simulink model "EcoSIM3_P2_C2"  (R2014b)
settings: Solver=ode1  SolverMode=SingleTasking  StartTime=0.0  StopTime=inf  FixedStep=0.01  RelTol=1e-3
PostLoadFcn:
  | %, if any(exist('dsrtsu_mdlpostloadfcn', 'file') == [2, 3, 6]), try dsrtsu_mdlpostloadfcn('Execute', bdroot); catch fprintf('Error in PostLoadFcn (dsrtsu_mdlpostloadfcn) for model "%s":\n %s\n', bdroot, lasterr); end, end,
InitFcn:
  | tic
  | %Startup_EcoSIM
values from neighbouring files (symbols this model uses):
  EngPwr = [0 5	10	15	20	25	30	35	40	45	50	55	60	65	70	75	80	85	90	95	100	105	110	115]    [Series_Maps.m]
  EngSpd = [0 477.4645 954.929 1909.858 2864.787 3819.716 4774.645 5729.574 6684.503]    [Series_Maps.m]
  EngTrq = [0	0	0	0	0	0	0	0	0	0	0	0	0	0	0	0	0	0	0	0	0	0	0	0 ... (first row only)    [Series_Maps.m]
  Power = [0 5 10 15 20 25 30]    [Series_Maps.m]
  Torque = [-50,-40,-30,-25,-20,-15,-10,-8,-6,-4,-2,0]    [Series_Maps.m]
undefined symbols (not defined in the file or in its folder): canChannel, Controls, DriveCycles, Driver, EM_EFF_MAP, EM_PwrLoss_MAP, Glbl, Plants, Veh_Dynamics
libraries: canmsglib x100, canlib x87, fl_lib x78, simulink x59, nesl_utility x40, sdl_lib x17, dspsigops x5, dspswit3 x3, dspstat3 x2, commnoisgen2 x1, dspfdesign x1
(part 6 of 15)

== system EcoSIM3_P2_C2/Supervisory Controller/Mode Operation/Accessory/ESS_Messages ==
  Bus Creator2 : BusCreator
  Constant : Constant
  Constant1 : Constant
  Constant2 : Constant
  Constant3 : Constant  Value=0
  Out1 : Outport
  wires:
  Constant/1 -> Bus Creator2/3  "hsc_bcm_leakage_ena"
  Constant2/1 -> Bus Creator2/1  "hsc_bcm_enable"
  Constant1/1 -> Bus Creator2/2  "hsc_bcm_mainc_close"
  Bus Creator2/1 -> Out1/1  "ESS_Signals_A123"
  Constant3/1 -> Bus Creator2/4  "hsc_bcm_epo"

== system EcoSIM3_P2_C2/Supervisory Controller/Mode Operation/Accessory/Engine Messages ==
  Bus Creator2 : BusCreator  Inputs=3
  Constant1 : Constant  Value=0
  Constant2 : Constant  Value=0
  Constant3 : Constant  Value=0
  Out1 : Outport
  wires:
  Constant1/1 -> Bus Creator2/1  "ICE_Torque_Request_Nm"
  Constant2/1 -> Bus Creator2/2  "Engine_On"
  Constant3/1 -> Bus Creator2/3  "Engine_Run"
  Bus Creator2/1 -> Out1/1  "ICE_Request"

== system EcoSIM3_P2_C2/Supervisory Controller/Mode Operation/Accessory/TM Messages ==
  Bus Creator3 : BusCreator  Inputs=3
  Constant1 : Constant  Value=0
  Constant3 : Constant  Value=0
  Constant6 : Constant  Value=0
  Out1 : Outport
  wires:
  Bus Creator3/1 -> Out1/1  "EM_Messages_Rhinehart"
  Constant1/1 -> Bus Creator3/1  "Inverter_Enable"
  Constant6/1 -> Bus Creator3/2  "Torque_Command"
  Constant3/1 -> Bus Creator3/3  "Rotation_Direction"

== system EcoSIM3_P2_C2/Supervisory Controller/Mode Operation/Accessory/Trans_Messages ==
  Bus Creator3 : BusCreator  Inputs=2
  Constant8 : Constant  Value=0
  Constant9 : Constant  Value=0
  Out1 : Outport
  wires:
  Constant9/1 -> Bus Creator3/2  "Gear_Request"
  Constant8/1 -> Bus Creator3/1  "Shift_Request"
  Bus Creator3/1 -> Out1/1  "Trans_Recieve"

== system EcoSIM3_P2_C2/Supervisory Controller/Mode Operation/Charging/BAS_Signals ==
  Bus Creator4 : BusCreator  Inputs=3
  Constant1 : Constant  Value=0
  Constant4 : Constant  Value=0
  Constant5 : Constant  Value=0
  Out1 : Outport
  wires:
  Constant5/1 -> Bus Creator4/3  "BAS_Mode_Request"
  Constant4/1 -> Bus Creator4/1  "BAS_Torque_Request_Nm"
  Bus Creator4/1 -> Out1/1  "BAS_SoftECU_Receive"
  Constant1/1 -> Bus Creator4/2  "BAS_Speed_Request"

== system EcoSIM3_P2_C2/Supervisory Controller/Mode Operation/Charging/DC//DC Enabled ==
  Bus Creator : BusCreator  Inputs=3
  Constant : Constant
  Constant1 : Constant  Value=12.8
  Constant2 : Constant
  Out1 : Outport
  wires:
  Constant/1 -> Bus Creator/1  "LowVoltEnablRq"
  Constant1/1 -> Bus Creator/2  "LwVltStpntCmnd"
  Constant2/1 -> Bus Creator/3  "PrplsnSysAtv"
  Bus Creator/1 -> Out1/1  "DC_DC"

== system EcoSIM3_P2_C2/Supervisory Controller/Mode Operation/Charging/EM_Signals ==
  Bus Creator3 : BusCreator  Inputs=3
  Constant1 : Constant  Value=0
  Constant3 : Constant  Value=0
  Constant6 : Constant  Value=0
  Out1 : Outport
  wires:
  Bus Creator3/1 -> Out1/1  "EM_Messages_Rhinehart"
  Constant6/1 -> Bus Creator3/2  "Torque_Command"
  Constant3/1 -> Bus Creator3/3  "Rotation_Direction"
  Constant1/1 -> Bus Creator3/1  "Inverter_Enable"

== system EcoSIM3_P2_C2/Supervisory Controller/Mode Operation/Charging/ESS_Messages ==
  From CAN : Inport
  Bus Creator1 : BusCreator
  Bus Selector1 : BusSelector  OutputSignals=ESS_Transmit.ESS_CAN_Out.BCM_Status.bcm_ready,ESS_Transmit.ESS_CAN_Out.BCM_Status.bcm_cpwr_cmd,ESS_Transmit.ESS_CAN_Out.BCM_Status.bcm_cpwr_mon,ESS_Transmit.ESS_CAN_Out.BCM_Data1.bcm_veh_mon,ESS_Transmit.ESS_CAN_Out.BCM_Status.bcm_mainc_stat
  Constant4 : Constant  Value=0
  Constant5 : Constant
  ESS Handshake : Stateflow chart  TreatAsAtomicUnit=on
  Out1 : Outport
  wires:
  Bus Selector1/5 -> ESS Handshake/5(bcm_mainc_stat)  "<bcm_mainc_stat>"
  ESS Handshake/3(hsc_bcm_leakage_ena) -> Bus Creator1/3  "hsc_bcm_leakage_ena"
  ESS Handshake/1(hsc_bcm_enable) -> Bus Creator1/1  "hsc_bcm_enable"
  From CAN/1 -> Bus Selector1/1
  Bus Selector1/3 -> ESS Handshake/3(bcm_cpwr_mon)  "<bcm_cpwr_mon>"
  Bus Selector1/2 -> ESS Handshake/2(bcm_cpwr_cmd)  "<bcm_cpwr_cmd>"
  Bus Selector1/1 -> ESS Handshake/1(bcm_ready)  "<bcm_ready>"
  ESS Handshake/2(hsc_bcm_mainc_close) -> Bus Creator1/2  "hsc_bcm_mainc_close"
  Bus Creator1/1 -> Out1/1  "ESS_Signals_A123"
  Bus Selector1/4 -> ESS Handshake/4(bcm_veh_mon)  "<bcm_veh_mon>"
  Constant4/1 -> Bus Creator1/4  "hsc_bcm_epo"
  Constant5/1 -> ESS Handshake/6(Veh_Start)

== system EcoSIM3_P2_C2/Supervisory Controller/Mode Operation/Charging/Engine Messages ==
  Bus Creator2 : BusCreator  Inputs=3
  Constant1 : Constant  Value=0
  Constant2 : Constant  Value=0
  Constant3 : Constant  Value=0
  Out1 : Outport
  wires:
  Constant1/1 -> Bus Creator2/1  "ICE_Torque_Request_Nm"
  Constant2/1 -> Bus Creator2/2  "Engine_On"
  Constant3/1 -> Bus Creator2/3  "Engine_Run"
  Bus Creator2/1 -> Out1/1  "ICE_Request"

== system EcoSIM3_P2_C2/Supervisory Controller/Mode Operation/Charging/Trans_Messages ==
  Bus Creator3 : BusCreator  Inputs=2
  Constant8 : Constant  Value=0
  Constant9 : Constant  Value=0
  Out1 : Outport
  wires:
  Constant9/1 -> Bus Creator3/2  "Gear_Request"
  Constant8/1 -> Bus Creator3/1  "Shift_Request"
  Bus Creator3/1 -> Out1/1  "Trans_Recieve"

== system EcoSIM3_P2_C2/Supervisory Controller/Mode Operation/EV/BAS_Signals ==
  Bus Creator4 : BusCreator  Inputs=3
  Constant1 : Constant  Value=0
  Constant4 : Constant  Value=0
  Constant5 : Constant
  Out1 : Outport
  wires:
  Constant5/1 -> Bus Creator4/3  "BAS_Mode_Request"
  Constant4/1 -> Bus Creator4/1  "BAS_Torque_Request_Nm"
  Bus Creator4/1 -> Out1/1  "BAS_SoftECU_Receive"
  Constant1/1 -> Bus Creator4/2  "BAS_Speed_Request"

== system EcoSIM3_P2_C2/Supervisory Controller/Mode Operation/EV/DC//DC Enabled ==
  Bus Creator : BusCreator  Inputs=3
  Constant : Constant
  Constant1 : Constant  Value=12.8
  Constant2 : Constant
  Out1 : Outport
  wires:
  Constant/1 -> Bus Creator/1  "LowVoltEnablRq"
  Constant1/1 -> Bus Creator/2  "LwVltStpntCmnd"
  Constant2/1 -> Bus Creator/3  "PrplsnSysAtv"
  Bus Creator/1 -> Out1/1  "DC_DC"

== system EcoSIM3_P2_C2/Supervisory Controller/Mode Operation/EV/ESS_Messages ==
  Bus Creator2 : BusCreator
  Constant : Constant
  Constant1 : Constant
  Constant2 : Constant
  Constant3 : Constant  Value=0
  Out1 : Outport
  wires:
  Constant/1 -> Bus Creator2/3  "hsc_bcm_leakage_ena"
  Constant2/1 -> Bus Creator2/1  "hsc_bcm_enable"
  Constant1/1 -> Bus Creator2/2  "hsc_bcm_mainc_close"
  Bus Creator2/1 -> Out1/1  "ESS_Signals_A123"
  Constant3/1 -> Bus Creator2/4  "hsc_bcm_epo"

== system EcoSIM3_P2_C2/Supervisory Controller/Mode Operation/EV/Engine Messages ==
  Bus Creator2 : BusCreator  Inputs=3
  Constant1 : Constant  Value=0
  Constant2 : Constant  Value=0
  Constant3 : Constant  Value=0
  Out1 : Outport
  wires:
  Constant1/1 -> Bus Creator2/1  "ICE_Torque_Request_Nm"
  Constant2/1 -> Bus Creator2/2  "Engine_On"
  Constant3/1 -> Bus Creator2/3  "Engine_Run"
  Bus Creator2/1 -> Out1/1  "ICE_Request"

== system EcoSIM3_P2_C2/Supervisory Controller/Mode Operation/EV/Trans_Messages ==
  Bus Creator3 : BusCreator  Inputs=2
  Constant8 : Constant  Value=0
  Constant9 : Constant
  Out1 : Outport
  wires:
  Constant9/1 -> Bus Creator3/2  "Gear_Request"
  Constant8/1 -> Bus Creator3/1  "Shift_Request"
  Bus Creator3/1 -> Out1/1  "Trans_Recieve"

== system EcoSIM3_P2_C2/Supervisory Controller/Mode Operation/Engine Only /BAS_Signals ==
  Bus Creator4 : BusCreator  Inputs=3
  Constant1 : Constant  Value=0
  Constant4 : Constant  Value=0
  Constant5 : Constant
  Out1 : Outport
  wires:
  Constant5/1 -> Bus Creator4/3  "BAS_Mode_Request"
  Constant4/1 -> Bus Creator4/1  "BAS_Torque_Request_Nm"
  Bus Creator4/1 -> Out1/1  "BAS_SoftECU_Receive"
  Constant1/1 -> Bus Creator4/2  "BAS_Speed_Request"

== system EcoSIM3_P2_C2/Supervisory Controller/Mode Operation/Engine Only /DC//DC Enabled ==
  Bus Creator : BusCreator  Inputs=3
  Constant : Constant
  Constant1 : Constant  Value=12.8
  Constant2 : Constant
  Out1 : Outport
  wires:
  Constant/1 -> Bus Creator/1  "LowVoltEnablRq"
  Constant1/1 -> Bus Creator/2  "LwVltStpntCmnd"
  Constant2/1 -> Bus Creator/3  "PrplsnSysAtv"
  Bus Creator/1 -> Out1/1  "DC_DC"

== system EcoSIM3_P2_C2/Supervisory Controller/Mode Operation/Engine Only /ESS_Messages ==
  Bus Creator2 : BusCreator
  Constant : Constant
  Constant1 : Constant
  Constant2 : Constant
  Constant3 : Constant  Value=0
  Out1 : Outport
  wires:
  Constant/1 -> Bus Creator2/3  "hsc_bcm_leakage_ena"
  Constant2/1 -> Bus Creator2/1  "hsc_bcm_enable"
  Constant1/1 -> Bus Creator2/2  "hsc_bcm_mainc_close"
  Bus Creator2/1 -> Out1/1  "ESS_Signals_A123"
  Constant3/1 -> Bus Creator2/4  "hsc_bcm_epo"

== system EcoSIM3_P2_C2/Supervisory Controller/Mode Operation/Engine Only /Engine Messages ==
  Bus Creator2 : BusCreator  Inputs=3
  Constant1 : Constant  Value=0
  Constant2 : Constant
  Constant3 : Constant
  Out1 : Outport
  wires:
  Constant1/1 -> Bus Creator2/1  "ICE_Torque_Request_Nm"
  Constant2/1 -> Bus Creator2/2  "Engine_On"
  Constant3/1 -> Bus Creator2/3  "Engine_Run"
  Bus Creator2/1 -> Out1/1  "ICE_Request"

== system EcoSIM3_P2_C2/Supervisory Controller/Mode Operation/Engine Only /Subsystem ==
  From CAN : Inport
  Supervisory : Inport  Port=2
  Bus Selector : BusSelector  OutputSignals=Driver Torque Request
  Bus Selector1 : BusSelector  OutputSignals=Clutch_Transmission_SoftECU_Transmit.Clutch_Transmission_CAN_Out.Message_1.Actual_Gear,Vehicle_speed.Vehicle_Speed_meter_per_s
  Engine Torque Calc : Subsystem
  Gain : Gain  Gain=1/(2.77)
  Gear Shift Requested 1 : Subsystem
  "ICE_Torque " : Outport
  Shift Requested : Outport  Port=2
  "Gear Requested " : Outport  Port=3
  wires:
  Engine Torque Calc/1(Eng_T_Opt) -> Gain/1, Gear Shift Requested 1/3(ICE_Torque_CMD [Nm])
  From CAN/1 -> Bus Selector1/1
  Gear Shift Requested 1/1("Shift Requested ") -> Shift Requested/1
  Gear Shift Requested 1/2("Gear Requested ") -> "Gear Requested "/1
  Bus Selector/1 -> Engine Torque Calc/3(Torque Request)  "<Driver Torque Request>"
  Supervisory/1 -> Bus Selector/1
  Bus Selector1/2 -> Gear Shift Requested 1/2(Vehicle_Speed [m/s]), Engine Torque Calc/2(Vehicle Speed)  "<Vehicle_Speed_meter_per_s>"
  Bus Selector1/1 -> Engine Torque Calc/1(Gear), Gear Shift Requested 1/1("Current Gear ")  "<Actual_Gear>"
  Gain/1 -> "ICE_Torque "/1

== system EcoSIM3_P2_C2/Supervisory Controller/Mode Operation/Engine Only /TM Messages ==
  In1 : Inport
  Bus Creator2 : BusCreator  Inputs=3
  Bus Selector : BusSelector  OutputSignals=Driver Torque Request
  Constant1 : Constant  Value=0
  Constant2 : Constant
  Gain : Gain  Gain=1/(2.77*2.77)
  Out1 : Outport
  wires:
  Gain/1 -> Bus Creator2/2  "Torque_Command"
  Constant1/1 -> Bus Creator2/3  "Rotation_Direction"
  Constant2/1 -> Bus Creator2/1  "Inverter_Enable"
  Bus Selector/1 -> Gain/1  "<Driver Torque Request>"
  Bus Creator2/1 -> Out1/1  "EM_Messages_Rhinehart"
  In1/1 -> Bus Selector/1

== system EcoSIM3_P2_C2/Supervisory Controller/Mode Operation/Engine Start /DC//DC Enabled ==
  Bus Creator : BusCreator  Inputs=3
  Constant : Constant
  Constant1 : Constant  Value=12.8
  Constant2 : Constant
  Out1 : Outport
  wires:
  Constant/1 -> Bus Creator/1  "LowVoltEnablRq"
  Constant1/1 -> Bus Creator/2  "LwVltStpntCmnd"
  Constant2/1 -> Bus Creator/3  "PrplsnSysAtv"
  Bus Creator/1 -> Out1/1  "DC_DC"

== system EcoSIM3_P2_C2/Supervisory Controller/Mode Operation/Engine Start /ESS_Messages ==
  Bus Creator2 : BusCreator
  Constant : Constant
  Constant1 : Constant
  Constant2 : Constant
  Constant3 : Constant  Value=0
  Out1 : Outport
  wires:
  Constant/1 -> Bus Creator2/3  "hsc_bcm_leakage_ena"
  Constant2/1 -> Bus Creator2/1  "hsc_bcm_enable"
  Constant1/1 -> Bus Creator2/2  "hsc_bcm_mainc_close"
  Bus Creator2/1 -> Out1/1  "ESS_Signals_A123"
  Constant3/1 -> Bus Creator2/4  "hsc_bcm_epo"

== system EcoSIM3_P2_C2/Supervisory Controller/Mode Operation/Engine Start /TM Messages ==
  In1 : Inport
  Bus Creator2 : BusCreator  Inputs=3
  Bus Selector : BusSelector  OutputSignals=Driver Torque Request
  Constant1 : Constant  Value=0
  Constant2 : Constant
  Gain : Gain  Gain=1/(2.77*2.77)
  Out1 : Outport
  wires:
  Gain/1 -> Bus Creator2/2  "Torque_Command"
  Constant1/1 -> Bus Creator2/3  "Rotation_Direction"
  Constant2/1 -> Bus Creator2/1  "Inverter_Enable"
  Bus Selector/1 -> Gain/1  "<Driver Torque Request>"
  Bus Creator2/1 -> Out1/1  "EM_Messages_Rhinehart"
  In1/1 -> Bus Selector/1

== system EcoSIM3_P2_C2/Supervisory Controller/Mode Operation/Engine Start /Trans Messages ==
  Bus Creator6 : BusCreator  Inputs=2
  Constant3 : Constant
  Ground : Ground
  Out1 : Outport
  wires:
  Constant3/1 -> Bus Creator6/2  "Gear_Request"
  Bus Creator6/1 -> Out1/1  "Trans_Receive"
  Ground/1 -> Bus Creator6/1  "Shift_Request"

== system EcoSIM3_P2_C2/Supervisory Controller/Mode Operation/Limited EV/BAS_Signals ==
  Bus Creator4 : BusCreator  Inputs=3
  Constant1 : Constant  Value=0
  Constant4 : Constant  Value=0
  Constant5 : Constant
  Out1 : Outport
  wires:
  Constant5/1 -> Bus Creator4/3  "BAS_Mode_Request"
  Constant4/1 -> Bus Creator4/1  "BAS_Torque_Request_Nm"
  Bus Creator4/1 -> Out1/1  "BAS_SoftECU_Receive"
  Constant1/1 -> Bus Creator4/2  "BAS_Speed_Request"

== system EcoSIM3_P2_C2/Supervisory Controller/Mode Operation/Limited EV/DC//DC Enabled ==
  Bus Creator : BusCreator  Inputs=3
  Constant : Constant
  Constant1 : Constant  Value=12.8
  Constant2 : Constant
  Out1 : Outport
  wires:
  Constant/1 -> Bus Creator/1  "LowVoltEnablRq"
  Constant1/1 -> Bus Creator/2  "LwVltStpntCmnd"
  Constant2/1 -> Bus Creator/3  "PrplsnSysAtv"
  Bus Creator/1 -> Out1/1  "DC_DC"

== system EcoSIM3_P2_C2/Supervisory Controller/Mode Operation/Limited EV/ESS_Messages ==
  Bus Creator2 : BusCreator
  Constant : Constant
  Constant1 : Constant
  Constant2 : Constant
  Constant3 : Constant  Value=0
  Out1 : Outport
  wires:
  Constant/1 -> Bus Creator2/3  "hsc_bcm_leakage_ena"
  Constant2/1 -> Bus Creator2/1  "hsc_bcm_enable"
  Constant1/1 -> Bus Creator2/2  "hsc_bcm_mainc_close"
  Bus Creator2/1 -> Out1/1  "ESS_Signals_A123"
  Constant3/1 -> Bus Creator2/4  "hsc_bcm_epo"

== system EcoSIM3_P2_C2/Supervisory Controller/Mode Operation/Limited EV/Engine Messages ==
  Bus Creator2 : BusCreator  Inputs=3
  Constant1 : Constant  Value=0
  Constant2 : Constant  Value=0
  Constant3 : Constant  Value=0
  Out1 : Outport
  wires:
  Constant1/1 -> Bus Creator2/1  "ICE_Torque_Request_Nm"
  Constant2/1 -> Bus Creator2/2  "Engine_On"
  Constant3/1 -> Bus Creator2/3  "Engine_Run"
  Bus Creator2/1 -> Out1/1  "ICE_Request"

== system EcoSIM3_P2_C2/Supervisory Controller/Mode Operation/Limited EV/Inverter Temp Selection  ==
  note: or we can use this?
  note: This is taking in all of the inverter temperatures and outputing the highest one
  In1 : Inport
  Bus Selector : BusSelector  OutputSignals=EM_CAN_Out.M160_Temperature_Set_1.Module_A,EM_CAN_Out.M160_Temperature_Set_1.Module_B,EM_CAN_Out.M160_Temperature_Set_1.Module_C,EM_CAN_Out.M160_Temperature_Set_1.Gate_Driver_Board,EM_CAN_Out.M161_Temperature_Set_2.Control_Board_Temperature
  Maximum : dspstat3/Maximum  fcn=Value and Index  reset=None  InputProcessing=Columns as channels (frame based)  indexBase=One  operateOver=Each column  Dimension=1  colComp=on  operation=maximum  roiEnable=off  roiType=Rectangles  roiPortion=Entire ROI  roiOutput=Individual statistics for each ROI  roiFlag=off  accumDataTypeStr=Inherit: Same as product output  accumLastDataTypeStr=Inherit: Same as product output  roundingMode=Floor  overflowMode=off
  MinMax : MinMax  Function=max  Inputs=5
  Relational Operator{,1..3} (4 alike) : RelationalOperator  OutDataTypeStr=boolean
  Switch{,1..3} (4 alike) : Switch  Criteria=u2 > Threshold
  Out1 : Outport
  wires:
  In1/1 -> Bus Selector/1
  Bus Selector/1 -> Switch/1, Relational Operator/1  "<Module_A>"
  Bus Selector/2 -> Switch/3, Relational Operator/2  "<Module_B>"
  Bus Selector/3 -> Relational Operator1/1, Switch1/1  "<Module_C>"
  Bus Selector/4 -> Switch1/3, Relational Operator1/2  "<Gate_Driver_Board>"
  Relational Operator/1 -> Switch/2
  Switch/1 -> Switch3/1, Relational Operator3/1
  Relational Operator1/1 -> Switch1/2
  Bus Selector/5 -> Switch2/3, Relational Operator2/2  "<Control_Board_Temperature>"
  Switch1/1 -> Switch2/1, Relational Operator2/1
  Relational Operator2/1 -> Switch2/2
  Switch2/1 -> Switch3/3, Relational Operator3/2
  Relational Operator3/1 -> Switch3/2
  Switch3/1 -> Out1/1  "Inverter_Temp"

== system EcoSIM3_P2_C2/Supervisory Controller/Mode Operation/Limited EV/Temperature Limiting ==
  Torque Request : Inport
  "Motor Temperature " : Inport  Port=2
  "Battery Temperature " : Inport  Port=3
  "Inverter Temperature " : Inport  Port=4
  Battery Temperature 1 : InportShadow  Port=3
  Chart : Stateflow chart  TreatAsAtomicUnit=on
  Compare To Constant : simulink/Logic and Bit Operations/Compare To Constant  relop=>  const=100  OutDataTypeStr=boolean
  Compare To Constant1 : simulink/Logic and Bit Operations/Compare To Constant  relop=>  const=70  OutDataTypeStr=boolean
  Compare To Constant2 : simulink/Logic and Bit Operations/Compare To Constant  relop=>  const=50  OutDataTypeStr=boolean
  Inverter Temperature 1 : InportShadow  Port=4
  Motor Temperature 1 : InportShadow  Port=2
  Multiport Switch : MultiPortSwitch  Inputs=4
  Product : Product
  Product1 : Product
  Product2 : Product
  Switch : Switch  Criteria=u2 > Threshold
  Switch1 : Switch  Criteria=u2 > Threshold
  Switch2 : Switch  Criteria=u2 > Threshold
  Temperature Gain : Lookup_n-D  NumberOfTableDimensions=1  BreakpointsForDimension1=[0 90 100 150]  Table=[1 1 .8 0]  InternalRulePriority=Speed  RndMeth=Simplest  InputSameDT=on
  Temperature Gain1 : Lookup_n-D  NumberOfTableDimensions=1  BreakpointsForDimension1="[0 70 76  95]"  Table=[1 1 .8 0 ]  InternalRulePriority=Speed  RndMeth=Simplest  InputSameDT=on
  Temperature Gain2 : Lookup_n-D  NumberOfTableDimensions=1  BreakpointsForDimension1=[0 50 60]  Table=[1 1 0]  InternalRulePriority=Speed  RndMeth=Simplest  InputSameDT=on
  Temperature Gain3 : Lookup_n-D  NumberOfTableDimensions=1  BreakpointsForDimension1=[0 90 100 150]  Table=[1 1 .8 0]  InternalRulePriority=Speed  RndMeth=Simplest  InputSameDT=on
  Torque Request_1 : InportShadow
  Torque Request_2 : InportShadow
  Torque Request_3 : InportShadow
  Torque Command : Outport
  wires:
  Torque Request_1/1 -> Product1/2, Switch1/3
  Temperature Gain1/1 -> Product1/1
  "Motor Temperature "/1 -> Compare To Constant/1, Temperature Gain/1
  "Inverter Temperature "/1 -> Compare To Constant1/1, Temperature Gain1/1
  Temperature Gain/1 -> Product/2
  "Battery Temperature "/1 -> Temperature Gain2/1, Compare To Constant2/1
  Temperature Gain2/1 -> Product2/1
  Compare To Constant2/1 -> Switch2/2
  Torque Request_2/1 -> Switch2/3, Product2/2
  Product1/1 -> Switch1/1
  Compare To Constant1/1 -> Switch1/2
  Product2/1 -> Switch2/1
  Multiport Switch/1 -> Torque Command/1
  Chart/1(out) -> Multiport Switch/1
  Switch/1 -> Multiport Switch/2
  Switch2/1 -> Multiport Switch/4
  Switch1/1 -> Multiport Switch/3
  Torque Request_3/1 -> Multiport Switch/5
  Motor Temperature 1/1 -> Chart/1(EM)
  Inverter Temperature 1/1 -> Chart/2(Inverter)
  Battery Temperature 1/1 -> Chart/3(Battery)
  Compare To Constant/1 -> Switch/2
  Torque Request/1 -> Product/1, Switch/3
  Product/1 -> Switch/1

== system EcoSIM3_P2_C2/Supervisory Controller/Mode Operation/Limited EV/Trans_Messages ==
  Bus Creator3 : BusCreator  Inputs=2
  Constant8 : Constant  Value=0
  Constant9 : Constant
  Out1 : Outport
  wires:
  Constant9/1 -> Bus Creator3/2  "Gear_Request"
  Constant8/1 -> Bus Creator3/1  "Shift_Request"
  Bus Creator3/1 -> Out1/1  "Trans_Recieve"

== system EcoSIM3_P2_C2/Supervisory Controller/Mode Operation/Series/DC//DC Enabled ==
  Bus Creator : BusCreator  Inputs=3
  Constant : Constant
  Constant1 : Constant  Value=12.8
  Constant2 : Constant
  Out1 : Outport
  wires:
  Constant/1 -> Bus Creator/1  "LowVoltEnablRq"
  Constant1/1 -> Bus Creator/2  "LwVltStpntCmnd"
  Constant2/1 -> Bus Creator/3  "PrplsnSysAtv"
  Bus Creator/1 -> Out1/1  "DC_DC"

== system EcoSIM3_P2_C2/Supervisory Controller/Mode Operation/Series/ESS_Messages ==
  Bus Creator2 : BusCreator
  Constant : Constant
  Constant1 : Constant
  Constant2 : Constant
  Constant3 : Constant  Value=0
  Out1 : Outport
  wires:
  Constant3/1 -> Bus Creator2/4  "hsc_bcm_epo"
  Bus Creator2/1 -> Out1/1  "ESS_Signals_A123"
  Constant1/1 -> Bus Creator2/2  "hsc_bcm_mainc_close"
  Constant2/1 -> Bus Creator2/1  "hsc_bcm_enable"
  Constant/1 -> Bus Creator2/3  "hsc_bcm_leakage_ena"

== system EcoSIM3_P2_C2/Supervisory Controller/Mode Operation/Series/Series Torque Determination  ==
  note: BAS Speed in RPM
  Battery SOC : Inport
  BAS : Lookup_n-D  BreakpointsForDimension1=Power  BreakpointsForDimension2=Torque  Table=Speed'  InternalRulePriority=Speed  RndMeth=Simplest  InputSameDT=on
  Belt Ratio : Gain  Gain=1/2.7
  Belt Ratio1 : Gain  Gain=-1
  Bus Selector : BusSelector  OutputSignals=ESS_Transmit.ESS_CAN_Out.BCM_Status.bcm_soc
  Constant1 : Constant  Value=50
  Constant3 : Constant  Value=-40
  Constant7 : Constant  Value=-20
  Engine : Lookup_n-D  BreakpointsForDimension1=EngSpd  BreakpointsForDimension2=EngPwr  Table=EngTrq  ExtrapMethod=Clip  InternalRulePriority=Speed  RndMeth=Simplest  InputSameDT=on
  Gain : Gain  Gain=1/(2.77)
  Rad/sec to RPM1 : Gain  Gain=9.54929
  Rad/sec to RPM2 : Gain  Gain=9.54929
  SOC Control : Subsystem
  Scope2 : Scope
      settings: YMin=14.81481  YMax=214.81481  SaveName=ScopeData7
  Terminator : Terminator
  BAS Speed : Outport
  Engine Torque : Outport  Port=2
  wires:
  BAS/1 -> Belt Ratio/1, Rad/sec to RPM2/1  "BAS_Speed_Request"
  Belt Ratio1/1 -> Engine/2
  Constant7/1 -> BAS/1, Belt Ratio1/1  "power [kW]"
  Engine/1 -> Scope2/1, Gain/1
  Constant3/1 -> BAS/2  "BAS_Torque_Request_Nm"
  Belt Ratio/1 -> Rad/sec to RPM1/1
  Gain/1 -> Engine Torque/1  "ICE_Torque_Request_Nm"
  Rad/sec to RPM1/1 -> Engine/1  "BAS_Speed_Request"
  Battery SOC/1 -> Bus Selector/1
  Constant1/1 -> SOC Control/2(SOC Target)
  Bus Selector/1 -> SOC Control/1(Battery SOC)  "<bcm_soc>"
  Rad/sec to RPM2/1 -> BAS Speed/1
  SOC Control/1(Power Request) -> Terminator/1

== system EcoSIM3_P2_C2/Supervisory Controller/Mode Operation/Series/Trans_Messages ==
  Bus Creator3 : BusCreator  Inputs=2
  Constant8 : Constant  Value=0
  Constant9 : Constant  Value=0
  Out1 : Outport
  wires:
  Constant9/1 -> Bus Creator3/2  "Gear_Request"
  Constant8/1 -> Bus Creator3/1  "Shift_Request"
  Bus Creator3/1 -> Out1/1  "Trans_Recieve"

== system EcoSIM3_P2_C2/Supervisory Controller/Mode Operation/Shutdown/BAS_Signals ==
  Bus Creator4 : BusCreator  Inputs=3
  Constant1 : Constant  Value=0
  Constant4 : Constant  Value=0
  Constant5 : Constant  Value=0
  Out1 : Outport
  wires:
  Constant5/1 -> Bus Creator4/3  "BAS_Mode_Request"
  Constant4/1 -> Bus Creator4/1  "BAS_Torque_Request_Nm"
  Bus Creator4/1 -> Out1/1  "BAS_SoftECU_Receive"
  Constant1/1 -> Bus Creator4/2  "BAS_Speed_Request"

== system EcoSIM3_P2_C2/Supervisory Controller/Mode Operation/Shutdown/DC//DC Disabled ==
  Bus Creator : BusCreator  Inputs=3
  Constant : Constant  Value=0
  Constant1 : Constant  Value=0
  Constant2 : Constant  Value=0
  Out1 : Outport
  wires:
  Constant/1 -> Bus Creator/1  "LowVoltEnablRq"
  Constant1/1 -> Bus Creator/2  "LwVltStpntCmnd"
  Constant2/1 -> Bus Creator/3  "PrplsnSysAtv"
  Bus Creator/1 -> Out1/1  "DC_DC"

== system EcoSIM3_P2_C2/Supervisory Controller/Mode Operation/Shutdown/Engine Messages ==
  Bus Creator2 : BusCreator  Inputs=3
  Constant1 : Constant  Value=0
  Constant2 : Constant  Value=0
  Constant3 : Constant  Value=0
  Out1 : Outport
  wires:
  Constant1/1 -> Bus Creator2/1  "ICE_Torque_Request_Nm"
  Constant2/1 -> Bus Creator2/2  "Engine_On"
  Constant3/1 -> Bus Creator2/3  "Engine_Run"
  Bus Creator2/1 -> Out1/1  "ICE_Request"

== system EcoSIM3_P2_C2/Supervisory Controller/Mode Operation/Shutdown/Shutdown ==
  In1 : Inport
  Bus Creator2 : BusCreator
  Bus Selector1 : BusSelector  OutputSignals=ESS_Transmit.ESS_CAN_Out.BCM_Status.bcm_ready,ESS_Transmit.ESS_CAN_Out.BCM_Status.bcm_cpwr_cmd,ESS_Transmit.ESS_CAN_Out.BCM_Status.bcm_cpwr_mon,ESS_Transmit.ESS_CAN_Out.BCM_Data1.bcm_veh_mon,GM_Transmit.GMLAN_CAN_Out.PPEI_Platform_General_Status.SysPwrMd,ESS_Transmit.ESS_CAN_Out.BCM_Status.bcm_mainc_stat
  Constant3 : Constant  Value=0
  ESS Handshake : Stateflow chart  TreatAsAtomicUnit=on
  Out1 : Outport
  wires:
  Bus Creator2/1 -> Out1/1  "ESS_Signals_A123"
  ESS Handshake/2(hsc_bcm_mainc_close) -> Bus Creator2/2  "hsc_bcm_mainc_close"
  Bus Selector1/2 -> ESS Handshake/2(bcm_cpwr_cmd)  "<bcm_cpwr_cmd>"
  ESS Handshake/1(hsc_bcm_enable) -> Bus Creator2/1  "hsc_bcm_enable"
  ESS Handshake/3(hsc_bcm_leakage_ena) -> Bus Creator2/3  "hsc_bcm_leakage_ena"
  Bus Selector1/3 -> ESS Handshake/3(bcm_cpwr_mon)  "<bcm_cpwr_mon>"
  Bus Selector1/5 -> ESS Handshake/5(Veh_Start)  "<SysPwrMd>"
  In1/1 -> Bus Selector1/1
  Constant3/1 -> Bus Creator2/4  "hsc_bcm_epo"
  Bus Selector1/4 -> ESS Handshake/4(bcm_veh_mon)  "<bcm_veh_mon>"
  Bus Selector1/1 -> ESS Handshake/1(bcm_ready)  "<bcm_ready>"
  Bus Selector1/6 -> ESS Handshake/6(bcm_mainc_stat)  "<bcm_mainc_stat>"

== system EcoSIM3_P2_C2/Supervisory Controller/Mode Operation/Shutdown/Shutdown Complete ==
  In1 : Inport
  In2 : Inport  Port=2
  Bus Selector1 : BusSelector  OutputSignals=hsc_bcm_enable
  Compare To Zero : simulink/Logic and Bit Operations/Compare To Zero  relop===  OutDataTypeStr=boolean
  Compare To Zero1 : simulink/Logic and Bit Operations/Compare To Zero  relop===  OutDataTypeStr=boolean
  Constant2 : Constant  Value=0
  Constant4 : Constant  Value=-1
  Logical Operator : Logic  AllPortsSameDT=off  OutDataTypeStr=boolean
  Switch : Switch  Threshold=1
  Out1 : Outport
  wires:
  Logical Operator/1 -> Switch/2
  Constant4/1 -> Switch/1
  Switch/1 -> Out1/1  "Vehicle_Ready"
  Bus Selector1/1 -> Compare To Zero1/1  "<hsc_bcm_enable>"
  Compare To Zero1/1 -> Logical Operator/1
  Constant2/1 -> Switch/3
  In1/1 -> Bus Selector1/1
  In2/1 -> Compare To Zero/1
  Compare To Zero/1 -> Logical Operator/2

== system EcoSIM3_P2_C2/Supervisory Controller/Mode Operation/Shutdown/Trans_Messages ==
  Bus Creator3 : BusCreator  Inputs=2
  Constant8 : Constant  Value=0
  Constant9 : Constant
  Out1 : Outport
  wires:
  Constant9/1 -> Bus Creator3/2  "Gear_Request"
  Constant8/1 -> Bus Creator3/1  "Shift_Request"
  Bus Creator3/1 -> Out1/1  "Trans_Recieve"

== system EcoSIM3_P2_C2/Supervisory Controller/Mode Operation/Startup/BAS Start up ==
  In1 : Inport
  BAS Handshake : Stateflow chart  TreatAsAtomicUnit=on
  Bus Creator4 : BusCreator  Inputs=3
  Bus Selector : BusSelector  OutputSignals=BAS_Transmit.BAS_CAN_Out.Status_2.Fault_U,BAS_Transmit.BAS_CAN_Out.Status_2.Fault_V,BAS_Transmit.BAS_CAN_Out.Status_2.Fault_W,ESS_Transmit.ESS_CAN_Out.BCM_Status.bcm_mainc_stat
  Constant : Constant  Value=0
  Constant1 : Constant  Value=0
  Logical Operator : Logic  Operator=OR  Inputs=3  AllPortsSameDT=off  OutDataTypeStr=boolean
  Memory : Memory
  Out1 : Outport
  wires:
  In1/1 -> Bus Selector/1
  Constant/1 -> Bus Creator4/1  "BAS_Torque_Request_Nm"
  Bus Creator4/1 -> Out1/1  "BAS_SoftECU_Receive"
  BAS Handshake/1(BAS_Mode_Request) -> Bus Creator4/3  "BAS_Mode_Request"
  Bus Selector/1 -> Logical Operator/1  "<Fault_U>"
  Bus Selector/4 -> BAS Handshake/2(bcm_mainc_stat)  "<bcm_mainc_stat>"
  Memory/1 -> BAS Handshake/1(BAS_Fault_Status)
  Constant1/1 -> Bus Creator4/2  "BAS_Speed_Request"
  Logical Operator/1 -> Memory/1
  Bus Selector/2 -> Logical Operator/2  "<Fault_V>"
  Bus Selector/3 -> Logical Operator/3  "<Fault_W>"

== system EcoSIM3_P2_C2/Supervisory Controller/Mode Operation/Startup/Battery Start Up  ==
  CAN : Inport
  Bus Creator2 : BusCreator
  Bus Selector1 : BusSelector  OutputSignals=ESS_Transmit.ESS_CAN_Out.BCM_Status.bcm_ready,ESS_Transmit.ESS_CAN_Out.BCM_Status.bcm_cpwr_cmd,ESS_Transmit.ESS_CAN_Out.BCM_Status.bcm_cpwr_mon,ESS_Transmit.ESS_CAN_Out.BCM_Data1.bcm_veh_mon,ESS_Transmit.ESS_CAN_Out.BCM_Status.bcm_mainc_stat,GM_Transmit.GMLAN_CAN_Out.PPEI_Platform_General_Status.SysPwrMd
  Compare To Constant : simulink/Logic and Bit Operations/Compare To Constant  relop=>  const=0  OutDataTypeStr=boolean
  Constant : Constant  Value=0
  Data Type Conversion : DataTypeConversion  OutDataTypeStr=double
  ESS Handshake : Stateflow chart  TreatAsAtomicUnit=on
  Out1 : Outport
  wires:
  Bus Selector1/5 -> ESS Handshake/5(bcm_mainc_stat)  "<bcm_mainc_stat>"
  ESS Handshake/3(hsc_bcm_leakage_ena) -> Bus Creator2/3  "hsc_bcm_leakage_ena"
  ESS Handshake/1(hsc_bcm_enable) -> Bus Creator2/1  "hsc_bcm_enable"
  CAN/1 -> Bus Selector1/1
  Bus Selector1/3 -> ESS Handshake/3(bcm_cpwr_mon)  "<bcm_cpwr_mon>"
  Bus Selector1/2 -> ESS Handshake/2(bcm_cpwr_cmd)  "<bcm_cpwr_cmd>"
  Bus Selector1/1 -> ESS Handshake/1(bcm_ready)  "<bcm_ready>"
  ESS Handshake/2(hsc_bcm_mainc_close) -> Bus Creator2/2  "hsc_bcm_mainc_close"
  Bus Creator2/1 -> Out1/1  "ESS_Signals_A123"
  Bus Selector1/4 -> ESS Handshake/4(bcm_veh_mon)  "<bcm_veh_mon>"
  Constant/1 -> Bus Creator2/4  "hsc_bcm_epo"
  Bus Selector1/6 -> Compare To Constant/1  "<SysPwrMd>"
  Compare To Constant/1 -> Data Type Conversion/1
  Data Type Conversion/1 -> ESS Handshake/6(Veh_Start)

== system EcoSIM3_P2_C2/Supervisory Controller/Mode Operation/Startup/DC//DC Enabled ==
  Bus Creator : BusCreator  Inputs=3
  Constant : Constant
  Constant1 : Constant  Value=12.8
  Constant2 : Constant
  Out1 : Outport
  wires:
  Constant/1 -> Bus Creator/1  "LowVoltEnablRq"
  Constant1/1 -> Bus Creator/2  "LwVltStpntCmnd"
  Constant2/1 -> Bus Creator/3  "PrplsnSysAtv"
  Bus Creator/1 -> Out1/1  "DC_DC"

== system EcoSIM3_P2_C2/Supervisory Controller/Mode Operation/Startup/EM Start up ==
  In1 : Inport
  Bus Creator : BusCreator  Inputs=3
  Bus Selector : BusSelector  OutputSignals=ESS_Transmit.ESS_CAN_Out.BCM_Status.bcm_mainc_stat,EM_Transmit.EM_CAN_Out.M170_Internal_States.Inverter_Enable_Lockout
  Constant : Constant  Value=0
  EM Handshake : Stateflow chart  TreatAsAtomicUnit=on
  Memory1 : Memory  X0=1
  Memory2 : Memory  X0=1
  Rotation_Direction : Constant  Value=0
  Scope : Scope  NumInputPorts=2
      settings: YMin=-0.125~-5  YMax=1.125~5  SaveName=ScopeData2
  Out1 : Outport
  wires:
  In1/1 -> Bus Selector/1
  Bus Selector/1 -> Memory2/1  "<bcm_mainc_stat>"
  Bus Selector/2 -> Scope/1, Memory1/1  "<Inverter_Enable_Lockout>"
  EM Handshake/1(Inverter_Enable) -> Bus Creator/1  "Inverter_Enable"
  Bus Creator/1 -> Out1/1  "EM_Messages_Rhinehart"
  Constant/1 -> Bus Creator/2  "Torque_Command"
  Rotation_Direction/1 -> Bus Creator/3  "Rotation_Direction"
  Memory1/1 -> Scope/2, EM Handshake/2(Inverter_Enable_Lockout)
  Memory2/1 -> EM Handshake/1(bcm_mainc_stat)

== system EcoSIM3_P2_C2/Supervisory Controller/Mode Operation/Startup/Engine Messages ==
  Bus Creator2 : BusCreator  Inputs=3
  Constant1 : Constant  Value=0
  Constant2 : Constant  Value=0
  Constant3 : Constant  Value=0
  Out1 : Outport
  wires:
  Constant1/1 -> Bus Creator2/1  "ICE_Torque_Request_Nm"
  Constant2/1 -> Bus Creator2/2  "Engine_On"
  Constant3/1 -> Bus Creator2/3  "Engine_Run"
  Bus Creator2/1 -> Out1/1  "ICE_Request"

== system EcoSIM3_P2_C2/Supervisory Controller/Mode Operation/Startup/Start up overide  ==
  In1 : Inport
  Bus Creator : BusCreator  Inputs=5
  Bus Selector : BusSelector  OutputSignals=Alpha_percent,GM_Transmit.GMLAN_CAN_Out.PPEI_Brake_Apply_Status.BrkPdlPos,GM_Transmit.GM_Electrical_Out.PRNDL,GM_Transmit.GMLAN_CAN_Out.PPEI_Platform_General_Status.SysPwrMd,ESS_Transmit.ESS_CAN_Out.BCM_Status.bcm_mainc_stat
  Gain : Gain
  Gain1 : Gain
  Gain2 : Gain
  Out1 : Outport
  wires:
  In1/1 -> Bus Selector/1
  Bus Selector/4 -> Bus Creator/4  "<SysPwrMd>"
  Bus Selector/3 -> Gain2/1  "<PRNDL>"
  Gain2/1 -> Bus Creator/3  "PRNDL"
  Bus Selector/2 -> Gain1/1  "<BrkPdlPos>"
  Gain1/1 -> Bus Creator/2  "Beta_percentage"
  Bus Selector/1 -> Gain/1  "<Alpha_percent>"
  Gain/1 -> Bus Creator/1  "Alpha_percentage"
  Bus Creator/1 -> Out1/1
  Bus Selector/5 -> Bus Creator/5  "<bcm_mainc_stat>"

== system EcoSIM3_P2_C2/Supervisory Controller/Mode Operation/Startup/Trans_Messages ==
  Bus Creator3 : BusCreator  Inputs=2
  Constant8 : Constant  Value=0
  Constant9 : Constant
  Out1 : Outport
  wires:
  Constant9/1 -> Bus Creator3/2  "Gear_Request"
  Constant8/1 -> Bus Creator3/1  "Shift_Request"
  Bus Creator3/1 -> Out1/1  "Trans_Recieve"

== system EcoSIM3_P2_C2/Supervisory Controller/Mode Operation/Startup/Vehicle Start Up  ==
  note: should be syspwrmd
  In1 : Inport
  Bus Selector : BusSelector  OutputSignals=Alpha_percentage,Beta_percentage,PRNDL,SysPwrMd
  Check for Accelerator Pedal : simulink/Logic and Bit Operations/Compare To Constant  relop=<  const=3.0  OutDataTypeStr=boolean
  Check for Brake : simulink/Logic and Bit Operations/Compare To Constant  relop=>=  const=15  OutDataTypeStr=boolean
  Check for Contactors Closed : simulink/Logic and Bit Operations/Compare To Constant  Commented=on  relop===  const=1  OutDataTypeStr=boolean
  Check for Park : simulink/Logic and Bit Operations/Compare To Constant  relop===  const=1  OutDataTypeStr=boolean
  "Check for Start Request " : simulink/Logic and Bit Operations/Compare To Constant  relop=>  const=0  OutDataTypeStr=boolean
  Data Type Conversion : DataTypeConversion  OutDataTypeStr=double
  Display4 : Display  Commented=on
  Logical Operator : Logic  AllPortsSameDT=off  OutDataTypeStr=boolean
  Logical Operator1 : Logic  AllPortsSameDT=off  OutDataTypeStr=boolean
  Logical Operator2 : Logic  AllPortsSameDT=off  OutDataTypeStr=boolean
  Sample and Hold : dspsigops/Sample and Hold  trig=Rising edge  initCond=0  latchinput=off
  Start : Outport
  wires:
  Check for Brake/1 -> Logical Operator/1  "check_brake"
  Check for Park/1 -> Logical Operator/2  "check_prndl"
  Check for Accelerator Pedal/1 -> Logical Operator1/1  "check_acc_ped"
  Logical Operator/1 -> Logical Operator1/2  "C2"
  Logical Operator1/1 -> Logical Operator2/1
  "Check for Start Request "/1 -> Logical Operator2/2  "check_key"
  ? -> Check for Contactors Closed/1  "<bcm_mainc_stat>"
  In1/1 -> Bus Selector/1
  Bus Selector/1 -> Check for Accelerator Pedal/1  "<Alpha_percentage>"
  Bus Selector/2 -> Check for Brake/1  "<Beta_percentage>"
  Bus Selector/3 -> Check for Park/1  "<PRNDL>"
  Bus Selector/4 -> "Check for Start Request "/1  "<SysPwrMd>"
  Logical Operator2/1 -> Data Type Conversion/1  "C3"
  Check for Contactors Closed/1 -> Display4/1
  Data Type Conversion/1 -> Sample and Hold/Trigger, Sample and Hold/1
  Sample and Hold/1 -> Start/1  "Startup_Complete"

== system EcoSIM3_P2_C2/Supervisory Controller/Mode Selection /Limp Home Mode Selection  /Fault Counter ==
  In1 : Inport
  Constant : Constant  Value=0
  Counter : dspswit3/Counter  Direction=Up  CountEvent=Rising edge  CounterSize=User defined  MaxCount=3  InitialCount=0  Output=Count  HitValue=32  ResetInput=on  SamplesPerFrame=1  Ts=1  CntDtype=double  HitDtype=Logical
  Display1 : Display
  Sample and Hold1 : dspsigops/Sample and Hold  trig=Rising edge  initCond=0  latchinput=off
  Scope : Scope
      settings: YMin=-0.125  YMax=1.125  SaveName=ScopeData7
  Scope1 : Scope
      settings: YMin=-0.125  YMax=1.125  SaveName=ScopeData4
  Scope2 : Scope
      settings: YMin=-0.125  YMax=1.125  SaveName=ScopeData12
  Shutdown : Constant  Value=3
  Switch : Switch  Threshold=3
  Fault_Code : Outport
  wires:
  Switch/1 -> Fault_Code/1  "Fault_Code"
  Shutdown/1 -> Switch/1
  Counter/1 -> Scope/1, Switch/2
  Sample and Hold1/1 -> Scope2/1, Switch/3
  Constant/1 -> Counter/2
  In1/1 -> Scope1/1, Sample and Hold1/Trigger, Display1/1, Counter/1, Sample and Hold1/1

== system EcoSIM3_P2_C2/Supervisory Controller/PRNDL/Determine Gear/Subsystem ==
  PRNDL Position : Inport
  bcm_epo : Inport  Port=2
  Logical Operator2 : Logic  AllPortsSameDT=off  OutDataTypeStr=boolean
  Logical Operator3 : Logic  AllPortsSameDT=off  OutDataTypeStr=boolean
  NOT PARK : simulink/Logic and Bit Operations/Compare To Constant  relop=~=  const=1  OutDataTypeStr=boolean  ZeroCross=off
  PARK : simulink/Logic and Bit Operations/Compare To Constant  relop===  const=1  OutDataTypeStr=boolean  ZeroCross=off
  Force Neutral : Outport
  Force Park : Outport  Port=2
  wires:
  PRNDL Position/1 -> PARK/1, NOT PARK/1
  Logical Operator3/1 -> Force Park/1
  PARK/1 -> Logical Operator3/1
  Logical Operator2/1 -> Force Neutral/1
  NOT PARK/1 -> Logical Operator2/1
  bcm_epo/1 -> Logical Operator3/2, Logical Operator2/2

== system EcoSIM3_P2_C2/Supervisory Controller/PRNDL/Drive/Check BAS Limits ==
  In1 : Inport
  Out1 : Outport
  wires:
  In1/1 -> Out1/1

== system EcoSIM3_P2_C2/Supervisory Controller/PRNDL/Drive/Check EM Limits ==
  In1 : Inport
  Constant : Constant  Value=inf
  Constant1 : Constant  Value=-inf
  Saturation Dynamic : simulink/Discontinuities/Saturation Dynamic  OutMin=[]  OutMax=[]  OutDataTypeStr=Inherit: Same as second input  OutDataType=fixdt(1, 16)  OutScaling=2^-10  DoSatur=off
  Out1 : Outport
  wires:
  In1/1 -> Saturation Dynamic/2
  Saturation Dynamic/1 -> Out1/1  "Torque_Command"
  Constant/1 -> Saturation Dynamic/1
  Constant1/1 -> Saturation Dynamic/3

== system EcoSIM3_P2_C2/Supervisory Controller/PRNDL/Drive/Check Engine Limits ==
  In1 : Inport
  Out1 : Outport
  wires:
  In1/1 -> Out1/1

== system EcoSIM3_P2_C2/Supervisory Controller/PRNDL/Reverse/Check BAS Limits ==
  In1 : Inport
  Out1 : Outport
  wires:
  In1/1 -> Out1/1

== system EcoSIM3_P2_C2/Supervisory Controller/PRNDL/Reverse/Check EM Limits ==
  In1 : Inport
  Out1 : Outport
  wires:
  In1/1 -> Out1/1

== system EcoSIM3_P2_C2/Supervisory Controller/PRNDL/Reverse/Ensure Desired Rotation Direction ==
  EM Torque Req I [Nm] : Inport
  VSM State [-] : Inport  Port=2
  "Rotation Direction Status [-] " : Inport  Port=3
  Constant : Constant  Value=0
  Logical Operator : Logic  AllPortsSameDT=off  OutDataTypeStr=boolean
  Logical Operator1 : Logic  Operator=NOT  Inputs=1  AllPortsSameDT=off  OutDataTypeStr=boolean
  OFF : simulink/Logic and Bit Operations/Compare To Constant  relop===  const=0  OutDataTypeStr=boolean
  ON : Constant
  READY : simulink/Logic and Bit Operations/Compare To Constant  relop===  const=5  OutDataTypeStr=boolean
  REVERSE : simulink/Logic and Bit Operations/Compare To Constant  relop===  const=0  OutDataTypeStr=boolean
  Switch : Switch  Criteria=u2 > Threshold  Threshold=.5
  Switch1 : Switch  Criteria=u2 > Threshold  Threshold=.5
  Switch2 : Switch  Criteria=u2 > Threshold  Threshold=.5
  TOGGLE : Subsystem
  reverse : Constant  Value=0
  EM Torque Req O [Nm] : Outport
  Inverter Enable Req [-] : Outport  Port=2
  Rotation Direction Req [-] : Outport  Port=3
  wires:
  "Rotation Direction Status [-] "/1 -> REVERSE/1, Switch2/3
  Switch/1 -> EM Torque Req O [Nm]/1
  Constant/1 -> Switch/3
  EM Torque Req I [Nm]/1 -> Switch/1
  Logical Operator/1 -> Switch/2
  VSM State [-]/1 -> READY/1
  READY/1 -> Logical Operator/1
  OFF/1 -> Switch2/2
  reverse/1 -> Switch2/1
  Switch2/1 -> Rotation Direction Req [-]/1
  Switch1/1 -> Inverter Enable Req [-]/1, OFF/1
  Logical Operator1/1 -> TOGGLE/Enable, Switch1/2
  TOGGLE/1(Out1) -> Switch1/1
  REVERSE/1 -> Logical Operator/2, Logical Operator1/1
  ON/1 -> Switch1/3

== system EcoSIM3_P2_C2/Supervisory Controller/Supervisory_IO/VNT Kvaser/CAN Rx ==
  BAS : Subsystem
  Bus Creator : BusCreator  Inputs=7
  Clutch Transmission : Subsystem
  ESS : Subsystem
  Electric Motor : Subsystem
  Engine : Subsystem
  GCM : Subsystem
  GMLAN : Subsystem
  CAN_Rx : Outport
  wires:
  Bus Creator/1 -> CAN_Rx/1
  GMLAN/1(GM) -> Bus Creator/2
  BAS/1(BAS) -> Bus Creator/3
  Clutch Transmission/1(Trans) -> Bus Creator/4
  Engine/1(ICETransmit) -> Bus Creator/5
  ESS/1(ESSTransmit) -> Bus Creator/6
  Electric Motor/1(EMTransmit) -> Bus Creator/7
  GCM/1(FromGCM) -> Bus Creator/1

== system EcoSIM3_P2_C2/Supervisory Controller/Supervisory_IO/VNT Kvaser/CAN Tx ==
  CAN Tx : Inport
  ESS : Subsystem
  Eelctric Motor : Subsystem
  ICE_BAS_Trans : Subsystem
  Mode : Subsystem
  wires:
  CAN Tx/1 -> ESS/1(ESS), ICE_BAS_Trans/1(ICE_BAS_Trans), Mode/1(Mode), Eelctric Motor/1(EMTransmit)

== system EcoSIM3_P2_C2/Supervisory Controller/Supervisory_IO/VNT Kvaser/Electrical Rx ==
  Bus Creator : BusCreator  Inputs=5
  Bus Creator{1,4..6,9} (5 alike) : BusCreator  Inputs=2
  Bus Creator2 : BusCreator  Inputs=1
  Bus Creator3 : BusCreator  Inputs=6
  Bus Selector : BusSelector  OutputSignals=From_SoftECU.GM_Electrical_Out.Drive_Mode,From_SoftECU.GM_Electrical_Out.PRNDL,From_SoftECU.GM_Electrical_Out.Alpha_Low,From_SoftECU.GM_Electrical_Out.Alpha_High,From_SoftECU.GM_Electrical_Out.Key_State,From_SoftECU.ESS_Electrical_Out.chga_ena
  Ground{,1..7} (8 alike) : Ground
  Electrical_Rx : Outport
  wires:
  [VNT_Electrical_FromGCM] -> Bus Creator1/1
  [VNT_Electrical_From_SoftECU] -> Bus Creator1/2  "From_SoftECU"
  Bus Creator1/1 -> Bus Selector/1
  Bus Selector/1 -> Bus Creator/1  "<Drive_Mode>"
  Bus Selector/2 -> Bus Creator/2  "<PRNDL>"
  Bus Selector/3 -> Bus Creator/3  "<Alpha_Low>"
  Bus Selector/4 -> Bus Creator/4  "<Alpha_High>"
  Bus Selector/5 -> Bus Creator/5  "<Key_State>"
  Bus Selector/6 -> Bus Creator2/1  "<chga_ena>"
  Bus Creator/1 -> Bus Creator3/3  "GM_Electrical_Out"
  Bus Creator2/1 -> Bus Creator3/4  "ESS_Electrical_Out"
  Bus Creator3/1 -> Electrical_Rx/1  "Electrical_Rx"
  Ground/1 -> Bus Creator4/1  "Dummy1"
  Ground1/1 -> Bus Creator4/2  "Dummy2"
  Bus Creator4/1 -> Bus Creator3/5  "BAS_Electrical_Out"
  Ground3/1 -> Bus Creator5/2  "Dummy2"
  Ground2/1 -> Bus Creator5/1  "Dummy1"
  Bus Creator5/1 -> Bus Creator3/2  "Clutch_Transmission_Electrical_Out"
  Ground5/1 -> Bus Creator6/2  "Dummy2"
  Ground4/1 -> Bus Creator6/1  "Dummy1"
  Bus Creator6/1 -> Bus Creator3/6  "ICE_Electrical_Out"
  Ground7/1 -> Bus Creator9/2  "Dummy2"
  Ground6/1 -> Bus Creator9/1  "Dummy1"
  Bus Creator9/1 -> Bus Creator3/1  "EM_Electrical_Out"

== system EcoSIM3_P2_C2/Supervisory Controller/Supervisory_IO/VNT Kvaser/Electrical Tx ==
  Electrical Tx : Inport
  Bus Creator : BusCreator  Inputs=2
  Bus Selector : BusSelector  OutputSignals=PON,chga_wake
  tag scope: VNT_Electrical_FromMABx=global
  wires:
  Bus Creator/1 -> [VNT_Electrical_FromMABx]  "Supervisory_Electrical_Out"
  Bus Selector/2 -> Bus Creator/2  "<chga_wake>"
  Bus Selector/1 -> Bus Creator/1  "<PON>"
  Electrical Tx/1 -> Bus Selector/1

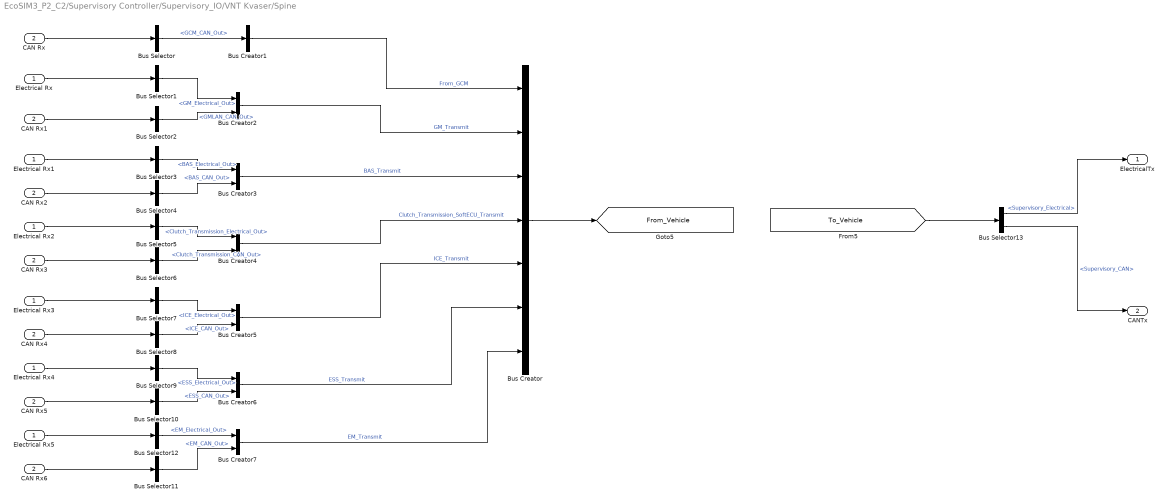
== system EcoSIM3_P2_C2/Supervisory Controller/Supervisory_IO/VNT Kvaser/Spine ==
  Electrical Rx : Inport
  CAN Rx : Inport  Port=2
  Bus Creator : BusCreator  Inputs=7
  Bus Creator1 : BusCreator  Inputs=1
  Bus Creator{2..7} (6 alike) : BusCreator  Inputs=2
  Bus Selector : BusSelector  OutputSignals=GCM_CAN_Out
  Bus Selector1 : BusSelector  OutputSignals=GM_Electrical_Out
  Bus Selector10 : BusSelector  OutputSignals=ESS_CAN_Out
  Bus Selector11 : BusSelector  OutputSignals=EM_CAN_Out
  Bus Selector12 : BusSelector  OutputSignals=EM_Electrical_Out
  Bus Selector13 : BusSelector  OutputSignals=Supervisory_Electrical,Supervisory_CAN
  Bus Selector2 : BusSelector  OutputSignals=GMLAN_CAN_Out
  Bus Selector3 : BusSelector  OutputSignals=BAS_Electrical_Out
  Bus Selector4 : BusSelector  OutputSignals=BAS_CAN_Out
  Bus Selector5 : BusSelector  OutputSignals=Clutch_Transmission_Electrical_Out
  Bus Selector6 : BusSelector  OutputSignals=Clutch_Transmission_CAN_Out
  Bus Selector7 : BusSelector  OutputSignals=ICE_Electrical_Out
  Bus Selector8 : BusSelector  OutputSignals=ICE_CAN_Out
  Bus Selector9 : BusSelector  OutputSignals=ESS_Electrical_Out
  CAN Rx{1..6} (6 alike) : InportShadow  Port=2
  Electrical Rx{1..5} (5 alike) : InportShadow
  ElectricalTx : Outport
  CANTx : Outport  Port=2
  tag scope: From_Vehicle=global
  wires:
  [To_Vehicle] -> Bus Selector13/1
  Bus Creator/1 -> [From_Vehicle]
  CAN Rx/1 -> Bus Selector/1
  Electrical Rx/1 -> Bus Selector1/1
  Bus Selector/1 -> Bus Creator1/1  "<GCM_CAN_Out>"
  Bus Creator1/1 -> Bus Creator/1  "From_GCM"
  CAN Rx1/1 -> Bus Selector2/1
  Bus Selector1/1 -> Bus Creator2/1  "<GM_Electrical_Out>"
  Bus Selector2/1 -> Bus Creator2/2  "<GMLAN_CAN_Out>"
  Bus Creator2/1 -> Bus Creator/2  "GM_Transmit"
  Electrical Rx1/1 -> Bus Selector3/1
  CAN Rx2/1 -> Bus Selector4/1
  Bus Selector3/1 -> Bus Creator3/1  "<BAS_Electrical_Out>"
  Bus Selector4/1 -> Bus Creator3/2  "<BAS_CAN_Out>"
  Bus Creator3/1 -> Bus Creator/3  "BAS_Transmit"
  Electrical Rx2/1 -> Bus Selector5/1
  CAN Rx3/1 -> Bus Selector6/1
  Bus Selector5/1 -> Bus Creator4/1  "<Clutch_Transmission_Electrical_Out>"
  Bus Selector6/1 -> Bus Creator4/2  "<Clutch_Transmission_CAN_Out>"
  Bus Creator4/1 -> Bus Creator/4  "Clutch_Transmission_SoftECU_Transmit"
  Electrical Rx3/1 -> Bus Selector7/1
  CAN Rx4/1 -> Bus Selector8/1
  Bus Selector7/1 -> Bus Creator5/1  "<ICE_Electrical_Out>"
  Bus Selector8/1 -> Bus Creator5/2  "<ICE_CAN_Out>"
  Bus Creator5/1 -> Bus Creator/5  "ICE_Transmit"
  Electrical Rx4/1 -> Bus Selector9/1
  CAN Rx5/1 -> Bus Selector10/1
  Bus Selector9/1 -> Bus Creator6/1  "<ESS_Electrical_Out>"
  Bus Selector10/1 -> Bus Creator6/2  "<ESS_CAN_Out>"
  Bus Creator6/1 -> Bus Creator/6  "ESS_Transmit"
  Electrical Rx5/1 -> Bus Selector12/1
  CAN Rx6/1 -> Bus Selector11/1
  Bus Selector12/1 -> Bus Creator7/1  "<EM_Electrical_Out>"
  Bus Selector11/1 -> Bus Creator7/2  "<EM_CAN_Out>"
  Bus Creator7/1 -> Bus Creator/7  "EM_Transmit"
  Bus Selector13/1 -> ElectricalTx/1  "<Supervisory_Electrical>"
  Bus Selector13/2 -> CANTx/1  "<Supervisory_CAN>"

== system EcoSIM3_P2_C2/Supervisory Controller/Supervisory_IO/VNT Vector/CAN Rx ==
  BAS : Subsystem
  Bus Creator : BusCreator  Inputs=7
  Clutch Transmission : Subsystem
  ESS : Subsystem
  Electric Motor : Subsystem
  Engine : Subsystem
  GCM : Subsystem
  GMLAN : Subsystem
  CAN_Rx : Outport
  wires:
  Bus Creator/1 -> CAN_Rx/1
  GMLAN/1(GM) -> Bus Creator/2
  BAS/1(BAS) -> Bus Creator/3
  Clutch Transmission/1(Trans) -> Bus Creator/4
  Engine/1(ICETransmit) -> Bus Creator/5
  ESS/1(ESSTransmit) -> Bus Creator/6
  Electric Motor/1(EMTransmit) -> Bus Creator/7
  GCM/1(FromGCM) -> Bus Creator/1

== system EcoSIM3_P2_C2/Supervisory Controller/Supervisory_IO/VNT Vector/CAN Tx ==
  CAN Tx : Inport
  ESS : Subsystem
  Eelctric Motor : Subsystem
  ICE_BAS_Trans : Subsystem
  Mode : Subsystem
  wires:
  CAN Tx/1 -> ESS/1(ESS), ICE_BAS_Trans/1(ICE_BAS_Trans), Mode/1(Mode), Eelctric Motor/1(EMTransmit)

== system EcoSIM3_P2_C2/Supervisory Controller/Supervisory_IO/VNT Vector/Electrical Rx ==
  Bus Creator : BusCreator  Inputs=5
  Bus Creator{1,4..6,9} (5 alike) : BusCreator  Inputs=2
  Bus Creator2 : BusCreator  Inputs=1
  Bus Creator3 : BusCreator  Inputs=6
  Bus Selector : BusSelector  OutputSignals=From_SoftECU.GM_Electrical_Out.Drive_Mode,From_SoftECU.GM_Electrical_Out.PRNDL,From_SoftECU.GM_Electrical_Out.Alpha_Low,From_SoftECU.GM_Electrical_Out.Alpha_High,From_SoftECU.GM_Electrical_Out.Key_State,From_SoftECU.ESS_Electrical_Out.chga_ena
  Ground{,1..7} (8 alike) : Ground
  Electrical_Rx : Outport
  wires:
  [VNT_Electrical_FromGCM] -> Bus Creator1/1
  [VNT_Electrical_From_SoftECU] -> Bus Creator1/2  "From_SoftECU"
  Bus Creator1/1 -> Bus Selector/1
  Bus Selector/1 -> Bus Creator/1  "<Drive_Mode>"
  Bus Selector/2 -> Bus Creator/2  "<PRNDL>"
  Bus Selector/3 -> Bus Creator/3  "<Alpha_Low>"
  Bus Selector/4 -> Bus Creator/4  "<Alpha_High>"
  Bus Selector/5 -> Bus Creator/5  "<Key_State>"
  Bus Selector/6 -> Bus Creator2/1  "<chga_ena>"
  Bus Creator/1 -> Bus Creator3/3  "GM_Electrical_Out"
  Bus Creator2/1 -> Bus Creator3/4  "ESS_Electrical_Out"
  Bus Creator3/1 -> Electrical_Rx/1  "Electrical_Rx"
  Ground/1 -> Bus Creator4/1  "Dummy1"
  Ground1/1 -> Bus Creator4/2  "Dummy2"
  Bus Creator4/1 -> Bus Creator3/5  "BAS_Electrical_Out"
  Ground3/1 -> Bus Creator5/2  "Dummy2"
  Ground2/1 -> Bus Creator5/1  "Dummy1"
  Bus Creator5/1 -> Bus Creator3/2  "Clutch_Transmission_Electrical_Out"
  Ground5/1 -> Bus Creator6/2  "Dummy2"
  Ground4/1 -> Bus Creator6/1  "Dummy1"
  Bus Creator6/1 -> Bus Creator3/6  "ICE_Electrical_Out"
  Ground7/1 -> Bus Creator9/2  "Dummy2"
  Ground6/1 -> Bus Creator9/1  "Dummy1"
  Bus Creator9/1 -> Bus Creator3/1  "EM_Electrical_Out"
